simulink model "step4_disturbance"  (R2025a)
settings: Solver=ode45  StartTime=0.0  StopTime=20  MaxStep=0.01  RelTol=1e-3
undefined symbols (not defined in the file or in its folder): A, B, F, K
libraries: SignalEditorBlockLib x1
settings Model: Creator=O M E N  LastModifiedBy=O M E N

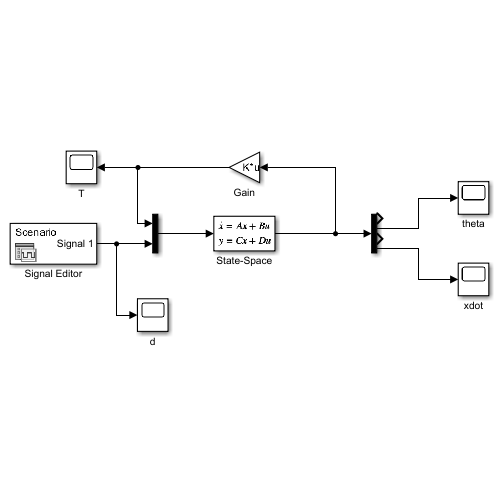
[thumbnail: Simulink's stored preview of the top-level diagram]
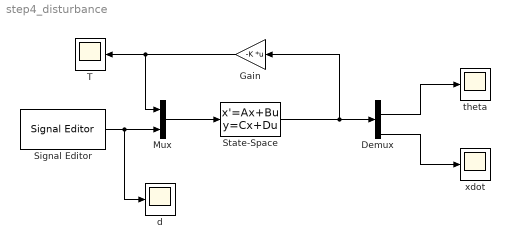
== system step4_disturbance ==
  Demux : Demux
  Gain : Gain  Gain=-K  Multiplication=Matrix(K*u)
  Mux : Mux  Inputs=2
  Signal Editor : SignalEditorBlockLib/Signal Editor  FileName=d_trapezoid.mat  ActiveScenario=Scenario  ActiveSignal=Signal 1  IsBus=off  OutputBusObjectStr=Bus: BusObject  SampleTime=0  ZeroCross=off  OutputAfterFinalValue=Setting to zero  Unit=inherit  PreserveSignalName=on  ApplySigPropsToAllScenarios=on  ApplySigPropsToAllSignals=off  SignalPropertySource=Dialog parameters
  State-Space : StateSpace  A=A  B=[B F]  C=eye(4)  D=zeros(4,2)  InitialCondition=[0; 0; 0; 0]
  T : Scope
      settings: Title=Control torque T(t)  ActiveDisplayYMinimum=-3.0690975343920019  ActiveDisplayYMaximum=11.898097533737634  YLabel="T  (N·m)"  DataLoggingVariableName=ScopeData2
  d : Scope
      settings: Title=Disturbance d(t)  ActiveDisplayYMinimum=-0.0012499999999999998  ActiveDisplayYMaximum=0.01125  YLabel="d  (m)"  DataLoggingVariableName=ScopeData3
  theta : Scope
      settings: Title=Tilt angle θ(t)  ActiveDisplayYMinimum=-0.0014361778362387047  ActiveDisplayYMaximum=0.0014361778372283518  YLabel="θ  (rad)"
  xdot : Scope
      settings: Title=Vehicle speed ẋ(t)  ActiveDisplayYMinimum=-0.14676890030256073  ActiveDisplayYMaximum=1.3209201027230468  YLabel="ẋ  (m/s)"
  wires:
  Mux/1 -> State-Space/1
  State-Space/1 -> Gain/1, Demux/1
  Demux/2 -> theta/1
  Demux/4 -> xdot/1
  Gain/1 -> T/1, Mux/1
  Signal Editor/1 -> d/1, Mux/2
